simulink model "BCex"  (Simulink 8.5)
settings: Solver=ode45  SolverMode=SingleTasking  StartTime=0.0  StopTime=0.3  RelTol=1e-3  AbsTol=1e-6
values from neighbouring files (symbols this model uses):
  tx = t-to    [ag1.m]
libraries: simulink x3, inputs x1, elements x1
settings Model: Creator=PC  LastModifiedBy=PC
settings DataIOCC: LimitDataPoints=off
settings OptimizationCC: BlockReduction=off  BooleanDataType=off  ExpressionDepthLimit=128
settings DebuggingCC: SaveWithParameterizedLinksMsg=none  SignalResolutionControl=TryResolveAllWithWarning  MultiTaskDSMMsg=warning  MultiTaskCondExecSysMsg=none  FcnCallInpInsideContextMsg=EnableAllAsError  StateNameClashWarn=none
settings HardwareCC: TargetUnknown=on

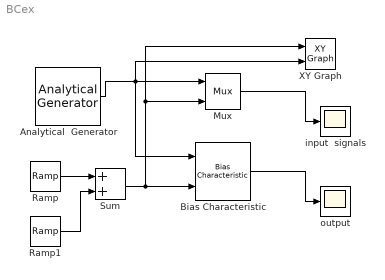
== system BCex ==
  Analytical  Generator : inputs/Analytical  Generator  y=5+5*cos(2*pi*60*tx)  to=0
  Bias Characteristic : elements/Bias Characteristic  BC=[ 0 0;15 15 ;30 0]  fs=60*20
  Mux : Mux  Inputs=2
  Ramp : simulink/Sources/Ramp  slope=100  start=0  X0=0
  Ramp1 : simulink/Sources/Ramp  slope=-200  start=0.15  X0=0
  Sum : Sum  SaturateOnIntegerOverflow=on  InputSameDT=on  OutDataTypeStr=Inherit: Same as first input
  XY Graph : simulink/Sinks/XY Graph  xmin=0  xmax=15  ymin=-1  ymax=10  st=1/(60*20)
  input  signals : Scope
      settings: TickLabels=on  TimeRange=0.3  YMax=30
  output : Scope
      settings: TickLabels=on  TimeRange=0.3  YMin=-0.1  YMax=1.1
  wires:
  Mux/1 -> input  signals/1
  Ramp1/1 -> Sum/2
  Ramp/1 -> Sum/1
  Sum/1 -> Bias Characteristic/2, Mux/2, XY Graph/1
  Bias Characteristic/1 -> output/1
  Analytical  Generator/1 -> Mux/1, XY Graph/2, Bias Characteristic/1
